simulink model "Kinematic_Model_Simulink"  (R2022a)
settings: Solver=ode14x  StartTime=0.0  StopTime=0.7  FixedStep=0.0005  RelTol=1e-3
values from neighbouring files (symbols this model uses):
  a_joint = 160/180*pi    (= 2.79252680319)    [Kinematic_Model_Activation.m]    (also in Kinematic_Model_sweep_double.m; Kinematic_Model_sweep_single.m)
  C_damping = 10    [Kinematic_Model_Activation.m]    (also in Kinematic_Model_sweep_double.m; Kinematic_Model_sweep_single.m = 100)
  g = [0;0;-9.81]    [Kinematic_Model_Activation.m]    (also in Kinematic_Model_sweep_double.m; Kinematic_Model_sweep_single.m)
  k_cable = 1200    [Kinematic_Model_Activation.m]    (also in Kinematic_Model_sweep_single.m)
  k_joint = 35    [Kinematic_Model_Activation.m]    (also in Kinematic_Model_sweep_double.m; Kinematic_Model_sweep_single.m)
  l_cable = sqrt(6)/4*l_leg*sin(a_joint/2)*(1 - delta)    [Kinematic_Model_Activation.m]    (also in Kinematic_Model_sweep_double.m; Kinematic_Model_sweep_single.m)
  l_leg = 0.3    [Kinematic_Model_Activation.m]    (also in Kinematic_Model_sweep_double.m; Kinematic_Model_sweep_single.m)
  m_bar = m_leg/2    (= 0.331383847657)    [Kinematic_Model_Activation.m]    (also in Kinematic_Model_sweep_double.m; Kinematic_Model_sweep_single.m)
  mu_k = 0.35    [Kinematic_Model_Activation.m]    (also in Kinematic_Model_sweep_double.m; Kinematic_Model_sweep_single.m)
  mu_s = 0.45    [Kinematic_Model_Activation.m]    (also in Kinematic_Model_sweep_double.m; Kinematic_Model_sweep_single.m)
  nu_s = 0.2    [Kinematic_Model_Activation.m]    (also in Kinematic_Model_sweep_double.m; Kinematic_Model_sweep_single.m)
  T_damping = 1    [Kinematic_Model_Activation.m]    (also in Kinematic_Model_sweep_double.m; Kinematic_Model_sweep_single.m)
(part 2 of 2)

== matlab function Kinematic_Model_Simulink/24 cables/cable 6--9 ==
  data: out_i output; E_cable output; out_j output; k_cable input; l_cable input; xi input; xj input; c input; vi input; vj input
function [out_i, E_cable, out_j]= cable(k_cable,l_cable,xi,xj,c,vi,vj)
% damp and D are initialized as zero
damp = 0;
D = 0;

% Node distance
x = xj-xi;
dist = norm(x);

% Only when the cable is in tension there is non-zero force and damping
if  dist-l_cable > 0
    D = dist-l_cable;
    v = vj - vi;
    damp = -c*dot(v,x)/dist^2;
end

% Forces on the end nodes
out_i = k_cable*D*(x)/dist - damp*(x);
out_j = -k_cable*D*(x)/dist + damp*(x);

% Energy stored in the cable
E_cable = 0.5*k_cable*D^2;
end

== matlab function Kinematic_Model_Simulink/24 cables/cable 1--2 ==
  data: out_i output; E_cable output; out_j output; k_cable input; l_cable input; xi input; xj input; c input; vi input; vj input
function [out_i, E_cable, out_j]= cable(k_cable,l_cable,xi,xj,c,vi,vj)
% damp and D are initialized as zero
damp = 0;
D = 0;

% Node distance
x = xj-xi;
dist = norm(x);

% Only when the cable is in tension there is non-zero force and damping
if  dist-l_cable > 0
    D = dist-l_cable;
    v = vj - vi;
    damp = -c*dot(v,x)/dist^2;
end

% Forces on the end nodes
out_i = k_cable*D*(x)/dist - damp*(x);
out_j = -k_cable*D*(x)/dist + damp*(x);

% Energy stored in the cable
E_cable = 0.5*k_cable*D^2;
end

== matlab function Kinematic_Model_Simulink/24 cables/cable 6--8 ==
  data: out_i output; E_cable output; out_j output; k_cable input; l_cable input; xi input; xj input; c input; vi input; vj input
function [out_i, E_cable, out_j]= cable(k_cable,l_cable,xi,xj,c,vi,vj)
% damp and D are initialized as zero
damp = 0;
D = 0;

% Node distance
x = xj-xi;
dist = norm(x);

% Only when the cable is in tension there is non-zero force and damping
if  dist-l_cable > 0
    D = dist-l_cable;
    v = vj - vi;
    damp = -c*dot(v,x)/dist^2;
end

% Forces on the end nodes
out_i = k_cable*D*(x)/dist - damp*(x);
out_j = -k_cable*D*(x)/dist + damp*(x);

% Energy stored in the cable
E_cable = 0.5*k_cable*D^2;
end

== matlab function Kinematic_Model_Simulink/24 cables/cable 6--10 ==
  data: out_i output; E_cable output; out_j output; k_cable input; l_cable input; xi input; xj input; c input; vi input; vj input
function [out_i, E_cable, out_j]= cable(k_cable,l_cable,xi,xj,c,vi,vj)
% damp and D are initialized as zero
damp = 0;
D = 0;

% Node distance
x = xj-xi;
dist = norm(x);

% Only when the cable is in tension there is non-zero force and damping
if  dist-l_cable > 0
    D = dist-l_cable;
    v = vj - vi;
    damp = -c*dot(v,x)/dist^2;
end

% Forces on the end nodes
out_i = k_cable*D*(x)/dist - damp*(x);
out_j = -k_cable*D*(x)/dist + damp*(x);

% Energy stored in the cable
E_cable = 0.5*k_cable*D^2;
end

== matlab function Kinematic_Model_Simulink/6 joints/Joint bar 2--8 ==
  data: xi input; alpha output; xj input; xk input; l input; x_joint output
function [alpha, x_joint]  = angle(xi, xj, xk, l)
%% Calculating the angle
d = norm(xi - xj); % Nodal distance
mag = (l^2-2*d^2)/l^2; % Term inside the inverse cosine to calculate the angle

if mag > -cos(160*pi/180)
    mag = -cos(160*pi/180);
    alpha = acos(mag);
else
    alpha = acos(mag);
end 

%% Plotting the Joint
% Distance from axis
d = l/2*cos(alpha/2);

% Vectors used for determination of the normal vector
nxi = transpose(xi);
nxj = transpose(xj);
nxk = transpose(xk);

% Normal vector of a plane created by a set of 2 parallel bars
normal = cross(nxi-nxj, nxi-nxk);
N = normal/norm(normal);

% Vector along the line between bar-connected nodes
x = nxj - nxi;
X = x/norm(x);

% Vector pointing outwards 
V = rotVec(X,N,-90);

% Position vector of the joint, to be used for plotting
x_joint = transpose(d*V + (nxj+nxi)/2);

end

== matlab function Kinematic_Model_Simulink/6 joints/Force bar 2--8 ==
  data: F_end_node_1 output; F_end_node_2 output; xi input; xj input; c input; vi input; vj input; m input; k_joint input; alpha input; l_bar input; a_joint input; g input; dt input
function [F_end_node_1, F_end_node_2]= Force(xi, xj, c, vi, vj, m, k_joint, alpha, l_bar, a_joint, g,dt)
% End node distance
x = xj - xi;
dist = norm(x);

% relative velocity of the two nodes w.r.t. each other
v = vj - vi;

% Torsion spring force and damping force
damp = -2*c*dot(x,v) / sqrt(dist^2*(l_bar^2 - dist^2)) * x/dist;
% Torsion spring force and damping force
if alpha < a_joint
    F_torsion = 1/2 * k_joint * (a_joint - alpha) / (cos(alpha/2)*l_bar/2);  
else
    F_torsion = - m/2*norm(v)/dt;
end

% Gravitational force
Fg_j = g/2;

% Calculation of the two parts of the torsion
F_end_node_1 = F_torsion *(-x)/dist - damp + Fg_j;
F_end_node_2 = F_torsion *x/dist + damp + Fg_j;

end

== matlab function Kinematic_Model_Simulink/6 joints/Angle bar 3--9 ==
  data: xi input; alpha output; xj input; xk input; l input; x_joint output
function [alpha, x_joint]  = angle(xi, xj, xk, l)
%% Calculating the angle
d = norm(xi - xj); % Nodal distance
mag = (l^2-2*d^2)/l^2; % Term inside the inverse cosine to calculate the angle

if mag > -cos(160*pi/180)
    mag = -cos(160*pi/180);
    alpha = acos(mag);
else
    alpha = acos(mag);
end 

%% Plotting the Joint
% Distance from axis
d = l/2*cos(alpha/2);

% Vectors used for determination of the normal vector
nxi = transpose(xi);
nxj = transpose(xj);
nxk = transpose(xk);

% Normal vector of a plane created by a set of 2 parallel bars
normal = cross(nxi-nxj, nxi-nxk);
N = normal/norm(normal);

% Vector along the line between bar-connected nodes
x = nxj - nxi;
X = x/norm(x);

% Vector pointing outwards 
V = rotVec(X,N,-90);

% Position vector of the joint, to be used for plotting
x_joint = transpose(d*V + (nxj+nxi)/2);

end

== matlab function Kinematic_Model_Simulink/6 joints/Force bar 3--9 ==
  data: F_end_node_1 output; F_end_node_2 output; xi input; xj input; c input; vi input; vj input; m input; k_joint input; alpha input; l_bar input; a_joint input; g input; dt input
function [F_end_node_1, F_end_node_2]= Force(xi, xj, c, vi, vj, m, k_joint, alpha, l_bar, a_joint, g,dt)
% End node distance
x = xj - xi;
dist = norm(x);

% relative velocity of the two nodes w.r.t. each other
v = vj - vi;

% Torsion spring force and damping force
damp = -2*c*dot(x,v) / sqrt(dist^2*(l_bar^2 - dist^2)) * x/dist;
% Torsion spring force and damping force
if alpha < a_joint
    F_torsion = 1/2 * k_joint * (a_joint - alpha) / (cos(alpha/2)*l_bar/2);  
else
    F_torsion = - m/2*norm(v)/dt;
end

% Gravitational force
Fg_j = g/2;

% Calculation of the two parts of the torsion
F_end_node_1 = F_torsion *(-x)/dist - damp + Fg_j;
F_end_node_2 = F_torsion *x/dist + damp + Fg_j;

end

== matlab function Kinematic_Model_Simulink/6 joints/Joint bar 4--10 ==
  data: xi input; alpha output; xj input; xk input; l input; x_joint output
function [alpha, x_joint]  = angle(xi, xj, xk, l)
%% Calculating the angle
d = norm(xi - xj); % Nodal distance
mag = (l^2-2*d^2)/l^2; % Term inside the inverse cosine to calculate the angle

if mag > -cos(160*pi/180)
    mag = -cos(160*pi/180);
    alpha = acos(mag);
else
    alpha = acos(mag);
end 

%% Plotting the Joint
% Distance from axis
d = l/2*cos(alpha/2);

% Vectors used for determination of the normal vector
nxi = transpose(xi);
nxj = transpose(xj);
nxk = transpose(xk);

% Normal vector of a plane created by a set of 2 parallel bars
normal = cross(nxi-nxj, nxi-nxk);
N = normal/norm(normal);

% Vector along the line between bar-connected nodes
x = nxj - nxi;
X = x/norm(x);

% Vector pointing outwards 
V = rotVec(X,N,-90);

% Position vector of the joint, to be used for plotting
x_joint = transpose(d*V + (nxj+nxi)/2);

end

== matlab function Kinematic_Model_Simulink/6 joints/Force bar 4--10 ==
  data: F_end_node_1 output; F_end_node_2 output; xi input; xj input; c input; vi input; vj input; m input; k_joint input; alpha input; l_bar input; a_joint input; g input; dt input
function [F_end_node_1, F_end_node_2]= Force(xi, xj, c, vi, vj, m, k_joint, alpha, l_bar, a_joint, g,dt)
% End node distance
x = xj - xi;
dist = norm(x);

% relative velocity of the two nodes w.r.t. each other
v = vj - vi;

% Torsion spring force and damping force
damp = -2*c*dot(x,v) / sqrt(dist^2*(l_bar^2 - dist^2)) * x/dist;
% Torsion spring force and damping force
if alpha < a_joint
    F_torsion = 1/2 * k_joint * (a_joint - alpha) / (cos(alpha/2)*l_bar/2);  
else
    F_torsion = - m/2*norm(v)/dt;
end

% Gravitational force
Fg_j = g/2;

% Calculation of the two parts of the torsion
F_end_node_1 = F_torsion *(-x)/dist - damp + Fg_j;
F_end_node_2 = F_torsion *x/dist + damp + Fg_j;

end

== matlab function Kinematic_Model_Simulink/6 joints/Joint bar 5--11 ==
  data: xi input; alpha output; xj input; xk input; l input; x_joint output
function [alpha, x_joint]  = angle(xi, xj, xk, l)
%% Calculating the angle
d = norm(xi - xj); % Nodal distance
mag = (l^2-2*d^2)/l^2; % Term inside the inverse cosine to calculate the angle

if mag > -cos(160*pi/180)
    mag = -cos(160*pi/180);
    alpha = acos(mag);
else
    alpha = acos(mag);
end 

%% Plotting the Joint
% Distance from axis
d = l/2*cos(alpha/2);

% Vectors used for determination of the normal vector
nxi = transpose(xi);
nxj = transpose(xj);
nxk = transpose(xk);

% Normal vector of a plane created by a set of 2 parallel bars
normal = cross(nxi-nxj, nxi-nxk);
N = normal/norm(normal);

% Vector along the line between bar-connected nodes
x = nxj - nxi;
X = x/norm(x);

% Vector pointing outwards 
V = rotVec(X,N,-90);

% Position vector of the joint, to be used for plotting
x_joint = transpose(d*V + (nxj+nxi)/2);

end

== matlab function Kinematic_Model_Simulink/6 joints/Force bar 5--11 ==
  data: F_end_node_1 output; F_end_node_2 output; xi input; xj input; c input; vi input; vj input; m input; k_joint input; alpha input; l_bar input; a_joint input; g input; dt input
function [F_end_node_1, F_end_node_2]= Force(xi, xj, c, vi, vj, m, k_joint, alpha, l_bar, a_joint, g,dt)
% End node distance
x = xj - xi;
dist = norm(x);

% relative velocity of the two nodes w.r.t. each other
v = vj - vi;

% Torsion spring force and damping force
damp = -2*c*dot(x,v) / sqrt(dist^2*(l_bar^2 - dist^2)) * x/dist;
% Torsion spring force and damping force
if alpha < a_joint
    F_torsion = 1/2 * k_joint * (a_joint - alpha) / (cos(alpha/2)*l_bar/2);  
else
    F_torsion = - m/2*norm(v)/dt;
end

% Gravitational force
Fg_j = g/2;

% Calculation of the two parts of the torsion
F_end_node_1 = F_torsion *(-x)/dist - damp + Fg_j;
F_end_node_2 = F_torsion *x/dist + damp + Fg_j;

end

== matlab function Kinematic_Model_Simulink/24 cables/cable 1--4 ==
  data: out_i output; E_cable output; out_j output; k_cable input; l_cable input; xi input; xj input; c input; vi input; vj input
function [out_i, E_cable, out_j]= cable(k_cable,l_cable,xi,xj,c,vi,vj)
% damp and D are initialized as zero
damp = 0;
D = 0;

% Node distance
x = xj-xi;
dist = norm(x);

% Only when the cable is in tension there is non-zero force and damping
if  dist-l_cable > 0
    D = dist-l_cable;
    v = vj - vi;
    damp = -c*dot(v,x)/dist^2;
end

% Forces on the end nodes
out_i = k_cable*D*(x)/dist - damp*(x);
out_j = -k_cable*D*(x)/dist + damp*(x);

% Energy stored in the cable
E_cable = 0.5*k_cable*D^2;
end

== matlab function Kinematic_Model_Simulink/6 joints/Joint bar 6--12 ==
  data: xi input; alpha output; xj input; xk input; l input; x_joint output
function [alpha, x_joint]  = angle(xi, xj, xk, l)
%% Calculating the angle
d = norm(xi - xj); % Nodal distance
mag = (l^2-2*d^2)/l^2; % Term inside the inverse cosine to calculate the angle

if mag > -cos(160*pi/180)
    mag = -cos(160*pi/180);
    alpha = acos(mag);
else
    alpha = acos(mag);
end 

%% Plotting the Joint
% Distance from axis
d = l/2*cos(alpha/2);

% Vectors used for determination of the normal vector
nxi = transpose(xi);
nxj = transpose(xj);
nxk = transpose(xk);

% Normal vector of a plane created by a set of 2 parallel bars
normal = cross(nxi-nxj, nxi-nxk);
N = normal/norm(normal);

% Vector along the line between bar-connected nodes
x = nxj - nxi;
X = x/norm(x);

% Vector pointing outwards 
V = rotVec(X,N,-90);

% Position vector of the joint, to be used for plotting
x_joint = transpose(d*V + (nxj+nxi)/2);

end

== matlab function Kinematic_Model_Simulink/6 joints/Force bar 6--12 ==
  data: xi input; xj input; c input; vi input; vj input; m input; F_end_node_1 output; F_end_node_2 output; k_joint input; alpha input; l_bar input; a_joint input; g input; dt input
function [F_end_node_1, F_end_node_2]= Force(xi, xj, c, vi, vj, m, k_joint, alpha, l_bar, a_joint, g,dt)
% End node distance
x = xj - xi;
dist = norm(x);

% relative velocity of the two nodes w.r.t. each other
v = vj - vi;

% Torsion spring force and damping force
damp = -2*c*dot(x,v) / sqrt(dist^2*(l_bar^2 - dist^2)) * x/dist;
% Torsion spring force and damping force
if alpha < a_joint
    F_torsion = 1/2 * k_joint * (a_joint - alpha) / (cos(alpha/2)*l_bar/2);  
else
    F_torsion = - m/2*norm(v)/dt;
end

% Gravitational force
Fg_j = g/2;

% Calculation of the two parts of the torsion
F_end_node_1 = F_torsion *(-x)/dist - damp + Fg_j;
F_end_node_2 = F_torsion *x/dist + damp + Fg_j;

end

== matlab function Kinematic_Model_Simulink/12 nodes /Leg 3--9/Friction 3--9 ==
  data: mu_k input; F_out_i output; mu_s input; nu_s input; m input; dt input; xi input; xj input; vi input; vj input; Fci input; Fcj input; F_out_j output; Fti input; Ftj input
function [F_out_i, F_out_j] = ground_friction(mu_k, mu_s, nu_s, m, dt, xi, xj, vi, vj, Fci, Fcj, Fti, Ftj)
F_fi = [0;0;0];
F_fj = [0;0;0];

F_ni = [0;0;0];
F_nj = [0;0;0];
%% Friction modelling: Stribeck
% Fc: Coulomb Friction
% Fs: Static Friction
% 
% If node i touches the ground the following if-loop will commence
if  xi(3) <= 0 && dt~= 0
    F_ni = [0; 0; -Fti(3)-Fci(3)] - [0; 0; m*vi(3)/dt]; % Normal force with the ground
    if F_ni(3) > 0
        F_c = mu_k*norm(F_ni); % Coulomb term
        F_s = mu_s*norm(F_ni); % Static term
        F_fi = -(F_c + (F_s-F_c)*exp(-(norm(vi)/nu_s)^2))*signum(vi) + F_ni; % Sum of frictional and normal forces on node i
    end
end
% If node j touches the ground the following if-loop will commence
if xj(3) <= 0 && dt~= 0
    F_nj = [0; 0; -Ftj(3)-Fcj(3)] - [0; 0; m*vj(3)/dt]; % Normal force with the ground
    if F_nj(3) > 0
        F_c = mu_k*norm(F_nj); % Coulomb term
        F_s = mu_s*norm(F_nj); % Static term
        F_fj = -(F_c + (F_s-F_c)*exp(-(norm(vj)/nu_s)^2))*signum(vj) + F_nj; % Sum of frictional and normal forces on node j
    end
end


F_out_i = Fci + Fti + F_fi;
F_out_j = Fcj + Ftj + F_fj;



end

== matlab function Kinematic_Model_Simulink/12 nodes /Leg 1--7/Friction 1--7 ==
  data: mu_k input; F_out_i output; mu_s input; nu_s input; m input; dt input; xi input; xj input; vi input; vj input; Fci input; Fcj input; F_out_j output; Fti input; Ftj input
function [F_out_i, F_out_j] = ground_friction(mu_k, mu_s, nu_s, m, dt, xi, xj, vi, vj, Fci, Fcj, Fti, Ftj)
F_fi = [0;0;0];
F_fj = [0;0;0];

F_ni = [0;0;0];
F_nj = [0;0;0];
%% Friction modelling: Stribeck
% Fc: Coulomb Friction
% Fs: Static Friction
% 
% If node i touches the ground the following if-loop will commence
if  xi(3) <= 0 && dt~= 0
    F_ni = [0; 0; -Fti(3)-Fci(3)] - [0; 0; m*vi(3)/dt]; % Normal force with the ground
    if F_ni(3) > 0
        F_c = mu_k*norm(F_ni); % Coulomb term
        F_s = mu_s*norm(F_ni); % Static term
        F_fi = -(F_c + (F_s-F_c)*exp(-(norm(vi)/nu_s)^2))*signum(vi) + F_ni; % Sum of frictional and normal forces on node i
    end
end
% If node j touches the ground the following if-loop will commence
if xj(3) <= 0 && dt~= 0
    F_nj = [0; 0; -Ftj(3)-Fcj(3)] - [0; 0; m*vj(3)/dt]; % Normal force with the ground
    if F_nj(3) > 0
        F_c = mu_k*norm(F_nj); % Coulomb term
        F_s = mu_s*norm(F_nj); % Static term
        F_fj = -(F_c + (F_s-F_c)*exp(-(norm(vj)/nu_s)^2))*signum(vj) + F_nj; % Sum of frictional and normal forces on node j
    end
end

F_out_i = Fci + Fti + F_fi;
F_out_j = Fcj + Ftj + F_fj;


end

== matlab function Kinematic_Model_Simulink/12 nodes /Leg 6-12/Friction 6--12 ==
  data: mu_k input; F_out_i output; mu_s input; nu_s input; m input; dt input; xi input; xj input; vi input; vj input; Fci input; Fcj input; F_out_j output; Fti input; Ftj input
function [F_out_i, F_out_j] = ground_friction(mu_k, mu_s, nu_s, m, dt, xi, xj, vi, vj, Fci, Fcj, Fti, Ftj)
F_fi = [0;0;0];
F_fj = [0;0;0];

F_ni = [0;0;0];
F_nj = [0;0;0];
%% Friction modelling: Stribeck
% Fc: Coulomb Friction
% Fs: Static Friction
% 
% If node i touches the ground the following if-loop will commence
if  xi(3) <= 0 && dt~= 0
    F_ni = [0; 0; -Fti(3)-Fci(3)] - [0; 0; m*vi(3)/dt]; % Normal force with the ground
    if F_ni(3) > 0
        F_c = mu_k*norm(F_ni); % Coulomb term
        F_s = mu_s*norm(F_ni); % Static term
        F_fi = -(F_c + (F_s-F_c)*exp(-(norm(vi)/nu_s)^2))*signum(vi) + F_ni; % Sum of frictional and normal forces on node i
        
    end
end
% If node j touches the ground the following if-loop will commence
if xj(3) <= 0 && dt~= 0
    F_nj = [0; 0; -Ftj(3)-Fcj(3)] - [0; 0; m*vj(3)/dt]; % Normal force with the ground
    if F_nj(3) > 0
        F_c = mu_k*norm(F_nj); % Coulomb term
        F_s = mu_s*norm(F_nj); % Static term
        F_fj = -(F_c + (F_s-F_c)*exp(-(norm(vj)/nu_s)^2))*signum(vj) + F_nj; % Sum of frictional and normal forces on node j
    end
end


F_out_i = Fci + Fti + F_fi;
F_out_j = Fcj + Ftj + F_fj;


end

== matlab function Kinematic_Model_Simulink/24 cables/cable 2--3 ==
  data: out_i output; E_cable output; out_j output; k_cable input; l_cable input; xi input; xj input; c input; vi input; vj input
function [out_i, E_cable, out_j]= cable(k_cable,l_cable,xi,xj,c,vi,vj)
% damp and D are initialized as zero
damp = 0;
D = 0;

% Node distance
x = xj-xi;
dist = norm(x);

% Only when the cable is in tension there is non-zero force and damping
if  dist-l_cable > 0
    D = dist-l_cable;
    v = vj - vi;
    damp = -c*dot(v,x)/dist^2;
end

% Forces on the end nodes
out_i = k_cable*D*(x)/dist - damp*(x);
out_j = -k_cable*D*(x)/dist + damp*(x);

% Energy stored in the cable
E_cable = 0.5*k_cable*D^2;
end

== matlab function Kinematic_Model_Simulink/12 nodes /Leg 5--11/Friction 5--11 ==
  data: mu_k input; F_out_i output; mu_s input; nu_s input; m input; dt input; xi input; xj input; vi input; vj input; Fci input; Fcj input; F_out_j output; Fti input; Ftj input
function [F_out_i, F_out_j] = ground_friction(mu_k, mu_s, nu_s, m, dt, xi, xj, vi, vj, Fci, Fcj, Fti, Ftj)
F_fi = [0;0;0];
F_fj = [0;0;0];

F_ni = [0;0;0];
F_nj = [0;0;0];
%% Friction modelling: Stribeck
% Fc: Coulomb Friction
% Fs: Static Friction
% 
% If node i touches the ground the following if-loop will commence
if  xi(3) <= 0 && dt~= 0
    F_ni = [0; 0; -Fti(3)-Fci(3)] - [0; 0; m*vi(3)/dt]; % Normal force with the ground
    if F_ni(3) > 0
        F_c = mu_k*norm(F_ni); % Coulomb term
        F_s = mu_s*norm(F_ni); % Static term
        F_fi = -(F_c + (F_s-F_c)*exp(-(norm(vi)/nu_s)^2))*signum(vi) + F_ni; % Sum of frictional and normal forces on node i
        
    end
end
% If node j touches the ground the following if-loop will commence
if xj(3) <= 0 && dt~= 0
    F_nj = [0; 0; -Ftj(3)-Fcj(3)] - [0; 0; m*vj(3)/dt]; % Normal force with the ground
    if F_nj(3) > 0
        F_c = mu_k*norm(F_nj); % Coulomb term
        F_s = mu_s*norm(F_nj); % Static term
        F_fj = -(F_c + (F_s-F_c)*exp(-(norm(vj)/nu_s)^2))*signum(vj) + F_nj; % Sum of frictional and normal forces on node j
    end
end




F_out_i = Fci + Fti + F_fi;
F_out_j = Fcj + Ftj + F_fj;



end
